simulink library "carnot"  (R2018b)
settings: Solver=VariableStepAuto  StartTime=0.0  StopTime=10.0  RelTol=1e-3
undefined symbols (not defined in the file or in its folder): A, A_earth, acol, Acol, ActPower1, ActPower2, ActPower3, Ad, Ad0, Ar, Au, Au0, Azimuth_Angle, B, Bd, Bd0, Br, Bu, Bu0, C, c1, c2, c3, c33, c4, c5, c6, CarnotCallbacks_Density, CarnotCallbacks_Enthalpy, CarnotCallbacks_Enthalpy2Temperature, CarnotCallbacks_Entropy, CarnotCallbacks_Evaporation_Enthalpy, CarnotCallbacks_GlobalMessageLevel, CarnotCallbacks_Grashof, CarnotCallbacks_Heat_Capacity, CarnotCallbacks_Kinematic_Viscosity, CarnotCallbacks_PMV_PPD, CarnotCallbacks_Prandtl, CarnotCallbacks_Saturation_Property, CarnotCallbacks_Saturation_Temperature, CarnotCallbacks_Saturation_Value_Water, CarnotCallbacks_Specific_Volume, CarnotCallbacks_Thermal_Conductivity, CarnotCallbacks_Vapour_Content, CarnotCallbacks_Vapour_Pressure, Cd, Cdl, Cr, Cu, Davies, Dd, DE_TRY2010_04_averageYear, delta_grd, density, DiameterLastPiece, dl, DPConstant, DPLinear, DPQuadratic, Dr ... (+59)
libraries: $bdroot x429, simulink x36, simulink_extras x12
(part 13 of 22)

== system carnot/Basic/Hydraulics/Grashof ==
  Twall : Inport
  Tinf : Inport  Port=2
  p : Inport  Port=3
  Fluid_Type : Inport  Port=4
  Fluid_Mix : Inport  Port=5
  dimension : Inport  Port=6
  SFunction : S-Function  FunctionName=grashofn  Parameters=DEBUGLEVEL,MAXTOTALMESSAGES,MAXCONSECUTIVEMESSAGES,WRITETOFILE,FILENAME  SFunctionDeploymentMode=off  EnableBusSupport=off
  Gr : Outport
  wires:
  SFunction/1 -> Gr/1
  Fluid_Type/1 -> SFunction/1
  Fluid_Mix/1 -> SFunction/2
  Twall/1 -> SFunction/3
  Tinf/1 -> SFunction/4
  p/1 -> SFunction/5
  dimension/1 -> SFunction/6

== system carnot/Basic/Hydraulics/Mix_T_Mdot ==
  THB1 : Inport
  THB2 : Inport  Port=2
  Add : Sum
  Bus Selector2 : BusSelector  OutputSignals=MassFlow
  Bus Selector3 : BusSelector  OutputSignals=MassFlow
  S-Function : S-Function  FunctionName=mix_temperature  Parameters=mixcalc  SFunctionDeploymentMode=off  EnableBusSupport=off
  select1 : Subsystem
  select2 : Subsystem
  T : Outport
  mdot : Outport  Port=2
  mix : Outport  Port=3
  wires:
  select2/1(Out1) -> S-Function/2
  select1/1(Out1) -> S-Function/1
  S-Function/1 -> T/1  "T"
  THB2/1 -> select2/1(In1), Bus Selector3/1
  S-Function/2 -> mix/1  "mix"
  THB1/1 -> select1/1(In1), Bus Selector2/1
  Bus Selector3/1 -> Add/2  "<MassFlow>"
  Bus Selector2/1 -> Add/1  "<MassFlow>"
  Add/1 -> mdot/1

== system carnot/Basic/Hydraulics/Prandtl ==
  T : Inport
  p : Inport  Port=2
  Fluid_Type : Inport  Port=3
  Fluid_Mix : Inport  Port=4
  SFunction : S-Function  FunctionName=prandtln  Parameters=DEBUGLEVEL,MAXTOTALMESSAGES,MAXCONSECUTIVEMESSAGES,WRITETOFILE,FILENAME  SFunctionDeploymentMode=off  EnableBusSupport=off
  Pr : Outport
  wires:
  SFunction/1 -> Pr/1
  T/1 -> SFunction/3
  p/1 -> SFunction/4
  Fluid_Type/1 -> SFunction/1
  Fluid_Mix/1 -> SFunction/2

== system carnot/Basic/Hydraulics/Reynolds ==
  T : Inport
  v : Inport  Port=2
  p : Inport  Port=3
  "fluid, mix" : Inport  Port=4
  dimension : Inport  Port=5
  Demux1 : Demux  Outputs=2
  Kinematic_Viscosity : $bdroot/Basic/Material_Properties/Kinematic_Viscosity  VariantControl=CarlibClassic  INPUTARGUMENTS=state variables (classic)  DEBUGLEVEL=WARNINGLEVEL  MAXTOTALMESSAGES=inf  MAXCONSECUTIVEMESSAGES=inf  WRITETOFILE=0  FILENAME='errors.txt'
  Product : Product  Inputs=/**  SaturateOnIntegerOverflow=on  InputSameDT=on  OutDataTypeStr=Inherit: Same as first input
  Re : Outport
  wires:
  Product/1 -> Re/1
  v/1 -> Product/2
  dimension/1 -> Product/3
  p/1 -> Kinematic_Viscosity/2
  T/1 -> Kinematic_Viscosity/1
  Demux1/1 -> Kinematic_Viscosity/3
  "fluid, mix"/1 -> Demux1/1
  Kinematic_Viscosity/1 -> Product/1
  Demux1/2 -> Kinematic_Viscosity/4

== system carnot/Basic/Hydraulics/ReynoldsTHB ==
  THB : Inport
  Diameter : Inport  Port=2
  Bus Selector : BusSelector  OutputSignals=Temperature,MassFlow,Pressure
  Bus Selector1 : BusSelector  OutputSignals=FluidType,FluidMix  OutputAsBus=on
  Bus Selector2 : BusSelector  OutputSignals=Temperature,Pressure
  Bus Selector3 : BusSelector  OutputSignals=FluidType,FluidMix  OutputAsBus=on
  Reynolds1 : $bdroot/Basic/Hydraulics/Reynolds
  Terminator : Terminator
  Velocity1 : $bdroot/Basic/Hydraulics/Velocity
  Re : Outport
  wires:
  Velocity1/1 -> Reynolds1/2
  Bus Selector/2 -> Velocity1/2  "<MassFlow>"
  Bus Selector/1 -> Velocity1/1  "<Temperature>"
  Bus Selector/3 -> Velocity1/3  "<Pressure>"
  Bus Selector1/1 -> Velocity1/4
  Bus Selector2/1 -> Reynolds1/1  "<Temperature>"
  Bus Selector3/1 -> Reynolds1/4
  Bus Selector2/2 -> Reynolds1/3  "<Pressure>"
  Velocity1/2 -> Terminator/1
  THB/1 -> Bus Selector/1, Bus Selector1/1, Bus Selector2/1, Bus Selector3/1
  Reynolds1/1 -> Re/1
  Diameter/1 -> Velocity1/5, Reynolds1/5

== system carnot/Basic/Hydraulics/THBCreator ==
  ID : Inport
  Temperature : Inport  Port=2
  MassFlow : Inport  Port=3
  Pressure : Inport  Port=4
  FluidType : Inport  Port=5
  FluidMix : Inport  Port=6
  FluidMix2 : Inport  Port=7
  FluidMix3 : Inport  Port=8
  DiameterLastPiece : Inport  Port=9
  DPConstant : Inport  Port=10
  DPLinear : Inport  Port=11
  DPQuadratic : Inport  Port=12
  HydraulicInductance : Inport  Port=13
  GeodeticHeight : Inport  Port=14
  BusCreator : BusCreator  Inputs=14  OutDataTypeStr=Bus: THB
  THB : Outport  OutDataTypeStr=Bus: THB
  wires:
  BusCreator/1 -> THB/1
  ID/1 -> BusCreator/1  "ID"
  Temperature/1 -> BusCreator/2  "Temperature"
  MassFlow/1 -> BusCreator/3  "MassFlow"
  Pressure/1 -> BusCreator/4  "Pressure"
  FluidType/1 -> BusCreator/5  "FluidType"
  FluidMix/1 -> BusCreator/6  "FluidMix"
  FluidMix2/1 -> BusCreator/7  "FluidMix2"
  FluidMix3/1 -> BusCreator/8  "FluidMix3"
  DiameterLastPiece/1 -> BusCreator/9  "DiameterLastPiece"
  DPConstant/1 -> BusCreator/10  "DPConstant"
  DPLinear/1 -> BusCreator/11  "DPLinear"
  DPQuadratic/1 -> BusCreator/12  "DPQuadratic"
  HydraulicInductance/1 -> BusCreator/13  "HydraulicInductance"
  GeodeticHeight/1 -> BusCreator/14  "GeodeticHeight"

== system carnot/Basic/Hydraulics/Velocity ==
  T : Inport
  mdot : Inport  Port=2
  p : Inport  Port=3
  "fluid, mix" : Inport  Port=4
  d : Inport  Port=5
  Demux1 : Demux  Outputs=2
  Density : $bdroot/Basic/Material_Properties/Density  VariantControl=CarlibClassic  INPUTARGUMENTS=state variables (classic)  DEBUGLEVEL=DEBUGLEVEL  MAXTOTALWARNINGS=inf  MAXCONSECUTIVEWARNINGS=inf  WRITETOFILE=0  FILENAME='errors.txt'
  Math Function : Math  Operator=square  SaturateOnIntegerOverflow=on
  Product : Product  Inputs=*//  SaturateOnIntegerOverflow=on  InputSameDT=on  OutDataTypeStr=Inherit: Same as first input
  quadratic : Gain  Gain=pi/4  SaturateOnIntegerOverflow=on  OutDataTypeStr=Inherit: Same as input  ParamDataTypeStr=Inherit: Same as input
  v : Outport
  density : Outport  Port=2
  wires:
  p/1 -> Density/2
  "fluid, mix"/1 -> Demux1/1
  Demux1/1 -> Density/3
  mdot/1 -> Product/1
  Demux1/2 -> Density/4
  T/1 -> Density/1
  Product/1 -> v/1
  d/1 -> Math Function/1
  Math Function/1 -> quadratic/1
  quadratic/1 -> Product/2
  Density/1 -> Product/3, density/1

== system carnot/Basic/Hydraulics/basic_THB ==
  Bus Creator : BusCreator  InitFcn=load THB.mat  Inputs=14  OutDataTypeStr=Bus: THB
  const1 : Constant  Value=hgt
  const2 : Constant  Value=mix2
  const21 : Constant  Value=ID  mask{mID=Pressure Drop from Massflow}
      mask prompts: mID "ID for pressure drop calculation"
      mask init:
      | ID = (mID-1)*10000+1;
      mask TypeOptions mID: No Pressure Drop | Pressure Drop from Massflow | Full Pressure Drop with Static Height
  const{22..23,30..31} (4 alike) : Constant  Value=0
  const24 : Constant  Value=t
  const25 : Constant  Value=mdot
  const26 : Constant  Value=p
  const27 : Constant  Value=fluid  mask{fluid=Water}
      mask TypeOptions fluid: Water | Air | Cotton Oil | Silicone Oil | Water-Glycol Mix | Tyfocor LS | Water (Constant 20°C) | Air (dry+ constant 20°C)
  const28 : Constant  Value=mix
  const29 : Constant  Value=dia
  const3 : Constant  Value=mix3
  THB : Outport
  wires:
  const28/1 -> Bus Creator/6  "FluidMix"
  const27/1 -> Bus Creator/5  "FluidType"
  const26/1 -> Bus Creator/4  "Pressure"
  const25/1 -> Bus Creator/3  "MassFlow"
  const24/1 -> Bus Creator/2  "Temperature"
  const21/1 -> Bus Creator/1  "ID"
  Bus Creator/1 -> THB/1
  const30/1 -> Bus Creator/10  "DPConstant"
  const29/1 -> Bus Creator/9  "DiameterLastPiece"
  const22/1 -> Bus Creator/11  "DPLinear"
  const23/1 -> Bus Creator/12  "DPQuadratic"
  const31/1 -> Bus Creator/13  "HydraulicInductance"
  const1/1 -> Bus Creator/14  "GeodeticHeight"
  const2/1 -> Bus Creator/7  "FluidMix2"
  const3/1 -> Bus Creator/8  "FluidMix3"

== system carnot/Basic/Hydraulics/basic_create_THB ==
  mdot : Inport
  T : Inport  Port=2
  THB_set_T : $bdroot/Source/Simple/THB_set_T
  THB_set_mdot : $bdroot/Source/Simple/THB_set_mdot
  basic_THB : $bdroot/Basic/Hydraulics/basic_THB  t=10  mdot=0  p=p  ID=No Pressure Drop  fluid=Water  mix=mix  mix2=mix2  mix3=mix3  dia=dia  hgt=hgt
  THB : Outport
  wires:
  T/1 -> THB_set_T/2
  THB_set_T/1 -> THB/1
  THB_set_mdot/1 -> THB_set_T/1
  mdot/1 -> THB_set_mdot/2
  basic_THB/1 -> THB_set_mdot/1

== system carnot/Basic/Material_Properties/AIV_WetBulbTemperature ==
  AIV : Inport
  AIV_selector : $bdroot/Outputs/AIV_selector  e1=off  e2=on  e3=off  e4=off  e5=off  e6=off  e7=off  e8=off  e9=off
  AIV_selector1 : $bdroot/Outputs/AIV_selector  e1=off  e2=off  e3=off  e4=off  e5=off  e6=off  e7=off  e8=on  e9=off
  AIV_selector2 : $bdroot/Outputs/AIV_selector  e1=off  e2=off  e3=off  e4=on  e5=off  e6=off  e7=off  e8=off  e9=off
  Bus Assignment : BusAssignment  AssignedSignals=Temperature,Pressure,FluidMix
  Constant_THB : $bdroot/Source/Simple/Constant_THB  t=20  mdot=0  p=1e5  mID=No Pressure Drop  fluid=Air  mix=0  mix2=0  mix3=0  dia=0.02  hgt=0
  THB_WetBulbTemperature : $bdroot/Basic/Material_Properties/THB_WetBulbTemperature
  WBT : Outport
  rel_hum : Outport  Port=2
  wires:
  THB_WetBulbTemperature/2 -> rel_hum/1
  Bus Assignment/1 -> THB_WetBulbTemperature/1
  Constant_THB/1 -> Bus Assignment/1
  AIV_selector1/1 -> Bus Assignment/3  "p"
  AIV_selector2/1 -> Bus Assignment/4  "mix"
  AIV_selector/1 -> Bus Assignment/2  "T"
  AIV/1 -> AIV_selector/1, AIV_selector2/1, AIV_selector1/1
  THB_WetBulbTemperature/1 -> WBT/1

== system carnot/Basic/Material_Properties/Density ==
  T : Inport
  p : Inport  Port=2
  Fluid_Type : Inport  Port=3
  Fluid_Mix : Inport  Port=4
  SFunction : S-Function  FunctionName=rhofluid  Parameters=DEBUGLEVEL-1,MAXTOTALWARNINGS,MAXCONSECUTIVEWARNINGS,WRITETOFILE,FILENAME  SFunctionDeploymentMode=off  EnableBusSupport=off
  density : Outport
  wires:
  SFunction/1 -> density/1
  T/1 -> SFunction/3
  p/1 -> SFunction/4
  Fluid_Type/1 -> SFunction/1
  Fluid_Mix/1 -> SFunction/2

== system carnot/Basic/Material_Properties/Enthalpy ==
  T : Inport
  p : Inport  Port=2
  Fluid_Type : Inport  Port=3
  Fluid_Mix : Inport  Port=4
  SFunction : S-Function  FunctionName=enthaflu  Parameters=DEBUGLEVEL,MAXTOTALMESSAGES,MAXCONSECUTIVEMESSAGES,WRITETOFILE,FILENAME  SFunctionDeploymentMode=off  EnableBusSupport=off
  enthalpy : Outport
  wires:
  SFunction/1 -> enthalpy/1
  T/1 -> SFunction/3
  p/1 -> SFunction/4
  Fluid_Type/1 -> SFunction/1
  Fluid_Mix/1 -> SFunction/2

== system carnot/Basic/Material_Properties/Enthalpy2Temperature ==
  enthalpy : Inport
  p : Inport  Port=2
  Fluid_Type : Inport  Port=3
  Fluid_Mix : Inport  Port=4
  SFunction : S-Function  FunctionName=enth2temp  Parameters=DEBUGLEVEL,MAXTOTALMESSAGES,MAXCONSECUTIVEMESSAGES,WRITETOFILE,FILENAME  SFunctionDeploymentMode=off  EnableBusSupport=off
  T : Outport
  wires:
  SFunction/1 -> T/1
  Fluid_Type/1 -> SFunction/1
  Fluid_Mix/1 -> SFunction/2
  enthalpy/1 -> SFunction/3
  p/1 -> SFunction/4

== system carnot/Basic/Material_Properties/Entropy ==
  T : Inport
  p : Inport  Port=2
  Fluid_Type : Inport  Port=3
  Fluid_Mix : Inport  Port=4
  SFunction : S-Function  FunctionName=entroflu  Parameters=DEBUGLEVEL,MAXTOTALMESSAGES,MAXCONSECUTIVEMESSAGES,WRITETOFILE,FILENAME  SFunctionDeploymentMode=off  EnableBusSupport=off
  entropy : Outport
  wires:
  SFunction/1 -> entropy/1
  T/1 -> SFunction/3
  p/1 -> SFunction/4
  Fluid_Type/1 -> SFunction/1
  Fluid_Mix/1 -> SFunction/2

== system carnot/Basic/Material_Properties/Evaporation_Enthalpy ==
  T : Inport
  p : Inport  Port=2
  Fluid_Type : Inport  Port=3
  Fluid_Mix : Inport  Port=4
  SFunction : S-Function  FunctionName=evapoent  Parameters=DEBUGLEVEL,MAXTOTALMESSAGES,MAXCONSECUTIVEMESSAGES,WRITETOFILE,FILENAME  SFunctionDeploymentMode=off  EnableBusSupport=off
  evap_enthalpy : Outport
  wires:
  SFunction/1 -> evap_enthalpy/1
  T/1 -> SFunction/3
  p/1 -> SFunction/4
  Fluid_Type/1 -> SFunction/1
  Fluid_Mix/1 -> SFunction/2

== system carnot/Basic/Material_Properties/Heat_Capacity ==
  T : Inport
  p : Inport  Port=2
  Fluid_Type : Inport  Port=3
  Fluid_Mix : Inport  Port=4
  SFunction : S-Function  FunctionName=capfluid  Parameters=DEBUGLEVEL-1,MAXTOTALWARNINGS,MAXCONSECUTIVEWARNINGS,WRITETOFILE,FILENAME  SFunctionDeploymentMode=off  EnableBusSupport=off
  cp : Outport
  wires:
  SFunction/1 -> cp/1
  T/1 -> SFunction/3
  p/1 -> SFunction/4
  Fluid_Type/1 -> SFunction/1
  Fluid_Mix/1 -> SFunction/2

== system carnot/Basic/Material_Properties/Input_Air ==
  Fluid_mix : Constant  Value=x
  Fluid_type : Constant  Value=2
  Temp : Constant  Value=T
  pres : Constant  Value=p
  Temperature : Outport
  Pressure : Outport  Port=2
  Fluid_type: air : Outport  Port=3
  absolute_humidity : Outport  Port=4
  wires:
  Fluid_mix/1 -> absolute_humidity/1
  Fluid_type/1 -> Fluid_type: air/1
  Temp/1 -> Temperature/1
  pres/1 -> Pressure/1

== system carnot/Basic/Material_Properties/Input_Cotton_Oil ==
  Fluid_mix : Constant  Value=0
  Fluid_type : Constant  Value=3
  Temp : Constant  Value=T
  pres : Constant  Value=p
  Temperature : Outport
  Pressure : Outport  Port=2
  Fluid_cotton_oil : Outport  Port=3
  mix : Outport  Port=4
  wires:
  pres/1 -> Pressure/1
  Temp/1 -> Temperature/1
  Fluid_type/1 -> Fluid_cotton_oil/1
  Fluid_mix/1 -> mix/1

== system carnot/Basic/Material_Properties/Input_Fluid ==
  Fluid_mix_ : Constant  Value=x
  Fluid_type_ : Constant  Value=fluid
  Temp : Constant  Value=T
  pres : Constant  Value=p
  Temperature : Outport
  Pressure : Outport  Port=2
  Fluid_type : Outport  Port=3
  Fluid_mix : Outport  Port=4
  wires:
  pres/1 -> Pressure/1
  Temp/1 -> Temperature/1
  Fluid_type_/1 -> Fluid_type/1
  Fluid_mix_/1 -> Fluid_mix/1

== system carnot/Basic/Material_Properties/Input_Silicon_Oil ==
  Fluid_mix : Constant  Value=0
  Fluid_type : Constant  Value=4
  Temp : Constant  Value=T
  pres : Constant  Value=p
  Temperature : Outport
  Pressure : Outport  Port=2
  Fluid_silicon_oil : Outport  Port=3
  mix : Outport  Port=4
  wires:
  Fluid_mix/1 -> mix/1
  Fluid_type/1 -> Fluid_silicon_oil/1
  Temp/1 -> Temperature/1
  pres/1 -> Pressure/1

== system carnot/Basic/Material_Properties/Input_Tyfocor_LS ==
  Fluid_mix : Constant  Value=0
  Fluid_type : Constant  Value=6
  Temp : Constant  Value=T
  pres : Constant  Value=p
  Temperature : Outport
  Pressure : Outport  Port=2
  Fluid_TyfocorLS : Outport  Port=3
  mix : Outport  Port=4
  wires:
  pres/1 -> Pressure/1
  Temp/1 -> Temperature/1
  Fluid_type/1 -> Fluid_TyfocorLS/1
  Fluid_mix/1 -> mix/1

== system carnot/Basic/Material_Properties/Input_Water ==
  Fluid_mix : Constant  Value=xd
  Fluid_type : Constant
  Temp : Constant  Value=T
  pres : Constant  Value=p
  Temperature : Outport
  Pressure : Outport  Port=2
  Fluid_type: water : Outport  Port=3
  vapour_content : Outport  Port=4
  wires:
  pres/1 -> Pressure/1
  Temp/1 -> Temperature/1
  Fluid_type/1 -> Fluid_type: water/1
  Fluid_mix/1 -> vapour_content/1

== system carnot/Basic/Material_Properties/Input_Water_Glycol ==
  Fluid_mix : Constant  Value=g
  Fluid_type : Constant  Value=5
  Temp : Constant  Value=T
  pres : Constant  Value=p
  Temperature : Outport
  Pressure : Outport  Port=2
  Fluid_type: water/glycol : Outport  Port=3
  "volume content of glycol " : Outport  Port=4
  wires:
  pres/1 -> Pressure/1
  Temp/1 -> Temperature/1
  Fluid_type/1 -> Fluid_type: water/glycol/1
  Fluid_mix/1 -> "volume content of glycol "/1

== system carnot/Basic/Material_Properties/Kinematic_Viscosity ==
  T : Inport
  p : Inport  Port=2
  Fluid_Type : Inport  Port=3
  Fluid_Mix : Inport  Port=4
  SFunction : S-Function  FunctionName=viscous  Parameters=DEBUGLEVEL,MAXTOTALMESSAGES,MAXCONSECUTIVEMESSAGES,WRITETOFILE,FILENAME  SFunctionDeploymentMode=off  EnableBusSupport=off
  visc : Outport
  wires:
  SFunction/1 -> visc/1
  T/1 -> SFunction/3
  p/1 -> SFunction/4
  Fluid_Type/1 -> SFunction/1
  Fluid_Mix/1 -> SFunction/2

== system carnot/Basic/Material_Properties/PhaseCheck ==
  THBin : Inport
  S-Function : S-Function  FunctionName=phasechk  SFunctionDeploymentMode=off  EnableBusSupport=off
  Selector : Selector  InputPortWidth=20  IndexOptions=Index vector (dialog)  Indices=[2:6]  OutputSizes=1
  THB2THV : $bdroot/Toolbox/THB2THV
  wires:
  Selector/1 -> S-Function/1
  THBin/1 -> THB2THV/1
  THB2THV/1 -> Selector/1

== system carnot/Basic/Material_Properties/RelHum2x ==
  note: RG      f · ps
      |  x  = ----  --------------
      |         RD     p - f · ps
      |
      | RG = 287.1 Nm/kgK (Gas Constant Air)
      | RD = 461.5 Nm/kgK (Gas Constant Water Vapour)
      | x absolute Humudity
      | f relative Humidity
      | pD partial pressure of water vapour
  T : Inport
  p : Inport  Port=2
  rel_hum : Inport  Port=3
  Product : Product  Inputs=*/  SaturateOnIntegerOverflow=on  InputSameDT=on  OutDataTypeStr=Inherit: Same as first input
  Product1 : Product  Inputs=*/  SaturateOnIntegerOverflow=on  InputSameDT=on  OutDataTypeStr=Inherit: Same as first input
  Saturation : Saturate  UpperLimit=inf  LowerLimit=0
  Sum : Sum  Inputs=-+  SaturateOnIntegerOverflow=on  InputSameDT=on  OutDataTypeStr=Inherit: Same as first input
  Vapour_Pressure : $bdroot/Basic/Material_Properties/Vapour_Pressure  VariantControl=CarlibClassic  INPUTARGUMENTS=state variables (classic)  DEBUGLEVEL=WARNINGLEVEL  MAXTOTALMESSAGES=inf  MAXCONSECUTIVEMESSAGES=inf  WRITETOFILE=0  FILENAME='errors.txt'
  mix : Constant  Value=0
  molar mass fraction : Gain  Gain=287.1/461.5  SaturateOnIntegerOverflow=on  OutDataTypeStr=Inherit: Same as input  ParamDataTypeStr=Inherit: Same as input
  p12 : Constant
  percent2absolute : Gain  Gain=0.01  SaturateOnIntegerOverflow=on  OutDataTypeStr=Inherit: Same as input  ParamDataTypeStr=Inherit: Same as input
  water : Constant
  x : Outport
  wires:
  p/1 -> Product/1
  Product/1 -> Sum/2
  Sum/1 -> Product1/2
  Product1/1 -> molar mass fraction/1
  T/1 -> Vapour_Pressure/1
  water/1 -> Vapour_Pressure/3
  p12/1 -> Vapour_Pressure/2
  mix/1 -> Vapour_Pressure/4
  Vapour_Pressure/1 -> Sum/1, Product1/1
  rel_hum/1 -> percent2absolute/1
  percent2absolute/1 -> Product/2
  molar mass fraction/1 -> Saturation/1
  Saturation/1 -> x/1

== system carnot/Basic/Material_Properties/Saturation_Property ==
  T : Inport
  p : Inport  Port=2
  Fluid_Type : Inport  Port=3
  Fluid_Mix : Inport  Port=4
  SFunction : S-Function  FunctionName=satprop  Parameters=PROPERTY, FLUIDPHASE, DEBUGLEVEL, MAXTOTALMESSAGES, MAXCONSECUTIVEMESSAGES, WRITETOFILE, FILENAME  SFunctionDeploymentMode=off  EnableBusSupport=off
  satprop : Outport
  wires:
  SFunction/1 -> satprop/1
  T/1 -> SFunction/3
  p/1 -> SFunction/4
  Fluid_Type/1 -> SFunction/1
  Fluid_Mix/1 -> SFunction/2

== system carnot/Basic/Material_Properties/Saturation_Temperature ==
  T : Inport
  p : Inport  Port=2
  Fluid_Type : Inport  Port=3
  Fluid_Mix : Inport  Port=4
  SFunction : S-Function  FunctionName=satutemp  Parameters=DEBUGLEVEL,MAXTOTALMESSAGES,MAXCONSECUTIVEMESSAGES,WRITETOFILE,FILENAME  SFunctionDeploymentMode=off  EnableBusSupport=off
  Tsat : Outport
  wires:
  SFunction/1 -> Tsat/1
  T/1 -> SFunction/3
  p/1 -> SFunction/4
  Fluid_Type/1 -> SFunction/1
  Fluid_Mix/1 -> SFunction/2

== system carnot/Basic/Material_Properties/Saturation_Value_Water ==
  T : Inport
  p : Inport  Port=2
  Fluid_Type : Inport  Port=3
  Fluid_Mix : Inport  Port=4
  property_id : Inport  Port=5
  SFunction : S-Function  FunctionName=satprop_vec  Parameters=DEBUGLEVEL,MAXTOTALMESSAGES,MAXCONSECUTIVEMESSAGES,WRITETOFILE,FILENAME  SFunctionDeploymentMode=off  EnableBusSupport=off
  saturation_vapour : Outport
  saturation_liquid : Outport  Port=2
  wires:
  SFunction/1 -> saturation_vapour/1
  SFunction/2 -> saturation_liquid/1
  T/1 -> SFunction/3
  p/1 -> SFunction/4
  Fluid_Type/1 -> SFunction/1
  Fluid_Mix/1 -> SFunction/2
  property_id/1 -> SFunction/5

== system carnot/Basic/Material_Properties/Specific_Volume ==
  T : Inport
  p : Inport  Port=2
  Fluid_Type : Inport  Port=3
  Fluid_Mix : Inport  Port=4
  SFunction : S-Function  FunctionName=specivol  Parameters=DEBUGLEVEL-1,MAXTOTALWARNINGS,MAXCONSECUTIVEWARNINGS,WRITETOFILE,FILENAME  SFunctionDeploymentMode=off  EnableBusSupport=off
  spec_vol : Outport
  wires:
  SFunction/1 -> spec_vol/1
  T/1 -> SFunction/3
  p/1 -> SFunction/4
  Fluid_Type/1 -> SFunction/1
  Fluid_Mix/1 -> SFunction/2

== system carnot/Basic/Material_Properties/THB_WetBulbTemperature ==
  THB_air : Inport
  Bus Selector : BusSelector  OutputSignals=Temperature,Pressure,FluidType,FluidMix
  Compare To Constant : simulink/Logic and Bit Operations/Compare To Constant  relop===  const=2  OutDataTypeStr=uint8  ZeroCross=off
  Constant : Constant
  Gain : Gain  Gain=100
  MinMax : MinMax  Inputs=2
  Product : Product  Inputs=*/  RndMeth=Zero
  Product1 : Product  RndMeth=Zero
  Product2 : Product  RndMeth=Zero
  Saturation : Saturate  UpperLimit=100  LowerLimit=0
  Vapour_Pressure1 : $bdroot/Basic/Material_Properties/Vapour_Pressure  VariantControl=CarlibClassic  INPUTARGUMENTS=state variables (classic)  DEBUGLEVEL=WARNINGLEVEL  MAXTOTALMESSAGES=inf  MAXCONSECUTIVEMESSAGES=inf  WRITETOFILE=0  FILENAME='errors.txt'
  Vapour_Pressure2 : $bdroot/Basic/Material_Properties/Vapour_Pressure  VariantControl=CarlibClassic  INPUTARGUMENTS=state variables (classic)  DEBUGLEVEL=WARNINGLEVEL  MAXTOTALMESSAGES=inf  MAXCONSECUTIVEMESSAGES=inf  WRITETOFILE=0  FILENAME='errors.txt'
  WBT Fcn of relHum+DBT : Lookup2D  RowIndex=[0,5,10,15,20,25,30,35,40,45,50,55,60,65,70,75,80,85,90,95,100]  ColumnIndex=[-6,-4,-2,0,2,4,6,8,10,12,14,16,18,20,22,24,26,28,30,32,34,36,38,40]  Table=reshape([-10.3,-10.1,-9.9,-9.3,-9.3,-8.9,-8.8,-8.8,-8.3,-8.2,-8.2,-7.7,-7.7,-7.7,-7.1,-7.1,-7.1,-6.6,-6.6,-6.0,-6,-8.3,-8.1,-7.9,-7.9,-7.8,-7.3,-7.3,-6.8,-6.8,-6.7,-6.2,-6.2,-5.7,-5.7,-5.6,-5.1,-5.1,-4.6,-4.6,-4.6,-4,-7.2,-6.9,-6.7,-6.4,-6.1,-5.9,-5.6,-5.3,-5.0,-4.8,-4.8,-4.2,-4.2,-3.7,-3.7,-3.1,-3.1,-2.6,-2.6,-2.6,-2,-5.6,-5.3,-5.0,-5.0,-4.4,-4.4,-3.9,-3.9,-3.3,-3.3,-2.8,-2.8,-2.2,-2.2,-1.7,-1.7,-1.1,-1.1,-0.6,-0.6,0,-4.5,-4.2,-3.9,-3.6,-3.0,-2.8,-2.4,-1.9,-1.9,-1.3,-1.3,-0.8,-0.6,-0.2,0.1,0.4,0.7,1.1,1.4,1.7,2,-3.4,-3.0,-2.7,-2.1,-1.6,-1.1,-1.0,-0.4,0.0,0.1,0.5,0.8,1.2,1.6,1.9,2.3,2.6,3.0,3.3,3.7,4,-1.9,-1.5,-1.1,-0.7,-0.3,0.1,0.5,0.9,1.3,1.8,2.2,2.6,3.0,3.4,3.8,4.1,4.5,4.9,5.3,5.6,6,-0.8,-0.4,0.1,0.6,1.1,1.5,2.0,2.5,2.9,3.4,3.8,4.3,4.7,5.1,5.6,6.0,6.4,6.8,7.2,7.6,8,0.3,0.8,1.4,1.9,2.5,3.0,3.5,4.0,4.5,5.0,5.5,6.0,6.5,6.9,7.4,7.8,8.3,8.7,9.2,9.6,10,1.4,2.1,2.7,3.3,3.9,4.4,5.0,5.6,6.1,6.6,7.2,7.7,8.2,8.7,9.2,9.7,10.2,10.6,11.1,11.6,12,2.6,3.2,3.9,4.6,5.2,5.8,6.5,7.1,7.7,8.2,8.8,9.4,9.9,10.5,11.0,11.5,12.0,12.5,13.0,13.5,14,3.7,4.4,5.1,5.9,6.6,7.3,7.9,8.6,9.2,9.9,10.5,11.1,11.7,12.2,12.8,13.4,13.9,14.5,15.0,15.5,16,4.7,5.5,6.3,7.1,7.9,8.6,9.4,10.1,10.8,11.5,12.1,12.8,13.4,14.0,14.6,15.2,15.8,16.4,16.9,17.5,18,5.7,6.6,7.5,8.4,9.2,10.0,10.8,11.6,12.3,13.1,13.8,14.5,15.1,15.8,16.4,17.1,17.7,18.3,18.9,19.4,20,6.7,7.7,8.7,9.6,10.5,11.4,12.2,13.1,13.9,14.6,15.4,16.1,16.9,17.6,18.2,18.9,19.6,20.2,20.8,21.4,22,7.7,8.8,9.8,10.8,11.8,12.8,13.7,14.6,15.4,16.2,17.0,17.8,18.6,19.3,20.1,20.8,21.4,22.1,22.7,23.4,24,8.6,9.8,11.0,12.1,13.1,14.1,15.1,16.0,17.0,17.8,18.7,19.5,20.3,21.1,21.9,22.6,23.3,24.0,24.7,25.4,26,9.6,10.8,12.1,13.3,14.4,15.5,16.5,17.5,18.5,19.4,20.3,21.2,22.1,22.9,23.7,24.5,25.2,25.9,26.6,27.3,28,10.4,11.8,13.2,14.4,15.7,16.8,17.9,19.0,20.0,21.0,22.0,22.9,23.8,24.7,25.5,26.3,27.1,27.8,28.6,29.3,30,11.3,12.8,14.3,15.6,16.9,18.2,19.4,20.5,21.6,22.6,23.6,24.6,25.5,26.4,27.3,28.2,29.0,29.8,30.5,31.3,32,12.1,13.8,15.3,16.8,18.2,19.5,20.8,22.0,23.1,24.2,25.3,26.3,27.3,28.2,29.1,30.0,30.9,31.7,32.5,33.3,34,12.9,14.7,16.4,18.0,19.5,20.9,22.2,23.5,24.7,25.9,27.0,28.0,29.0,30.0,31.0,31.9,32.8,33.6,34.4,35.2,36,13.7,15.7,17.5,19.1,20.7,22.2,23.6,25.0,26.3,27.5,28.6,29.7,30.8,31.8,32.8,33.7,34.7,35.5,36.4,37.2,38,14.5,16.6,18.5,20.3,22.0,23.6,25.1,26.5,27.8,29.1,30.3,31.5,32.6,33.6,34.6,35.6,36.6,37.5,38.3,39.2,40],21,24)  RndMeth=Nearest  LUTDesignDataSource=Matlab Workspace  LUTDesignUseExistingBP=off  LUTDesignAbsError=NaN
  WBT : Outport
  rel_hum : Outport  Port=2
  wires:
  Compare To Constant/1 -> Product1/2, Product2/2
  Product2/1 -> WBT/1
  Product1/1 -> rel_hum/1
  Saturation/1 -> Product1/1, WBT Fcn of relHum+DBT/1
  Gain/1 -> Saturation/1
  WBT Fcn of relHum+DBT/1 -> Product2/1
  Product/1 -> Gain/1
  MinMax/1 -> Product/1
  Vapour_Pressure2/1 -> Product/2, MinMax/2
  Vapour_Pressure1/1 -> MinMax/1
  Constant/1 -> Vapour_Pressure2/3, Vapour_Pressure2/4
  Bus Selector/1 -> Vapour_Pressure1/1, Vapour_Pressure2/1, WBT Fcn of relHum+DBT/2  "<Temperature>"
  Bus Selector/4 -> Vapour_Pressure1/4  "<FluidMix>"
  Bus Selector/3 -> Compare To Constant/1, Vapour_Pressure1/3  "<FluidType>"
  Bus Selector/2 -> Vapour_Pressure1/2, Vapour_Pressure2/2  "<Pressure>"
  THB_air/1 -> Bus Selector/1

== system carnot/Basic/Material_Properties/Temperature_Conductivity ==
  T : Inport
  p : Inport  Port=2
  Fluid_Type : Inport  Port=3
  Fluid_Mix : Inport  Port=4
  SFunction : S-Function  FunctionName=tempconduct  Parameters=DEBUGLEVEL,MAXTOTALMESSAGES,MAXCONSECUTIVEMESSAGES,WRITETOFILE,FILENAME  SFunctionDeploymentMode=off  EnableBusSupport=off
  Tcond : Outport
  wires:
  SFunction/1 -> Tcond/1
  T/1 -> SFunction/3
  p/1 -> SFunction/4
  Fluid_Type/1 -> SFunction/1
  Fluid_Mix/1 -> SFunction/2

== system carnot/Basic/Material_Properties/Thermal_Conductivity ==
  T : Inport
  p : Inport  Port=2
  Fluid_Type : Inport  Port=3
  Fluid_Mix : Inport  Port=4
  SFunction : S-Function  FunctionName=conduct  Parameters=DEBUGLEVEL,MAXTOTALMESSAGES,MAXCONSECUTIVEMESSAGES,WRITETOFILE,FILENAME  SFunctionDeploymentMode=off  EnableBusSupport=off
  cond : Outport
  wires:
  SFunction/1 -> cond/1
  T/1 -> SFunction/3
  p/1 -> SFunction/4
  Fluid_Type/1 -> SFunction/1
  Fluid_Mix/1 -> SFunction/2

== system carnot/Basic/Material_Properties/Vapour_Content ==
  T : Inport
  p : Inport  Port=2
  Fluid_Type : Inport  Port=3
  Fluid_Mix : Inport  Port=4
  value : Inport  Port=5
  SFunction : S-Function  FunctionName=vapocont  Parameters=PROPERTYTYPE, DEBUGLEVEL, MAXTOTALMESSAGES, MAXCONSECUTIVEMESSAGES,WRITETOFILE, FILENAME  SFunctionDeploymentMode=off  EnableBusSupport=off
  vapcont : Outport
  wires:
  SFunction/1 -> vapcont/1
  T/1 -> SFunction/3
  p/1 -> SFunction/4
  Fluid_Type/1 -> SFunction/1
  Fluid_Mix/1 -> SFunction/2
  value/1 -> SFunction/5

== system carnot/Basic/Material_Properties/Vapour_Pressure ==
  T : Inport
  p : Inport  Port=2
  Fluid_Type : Inport  Port=3
  Fluid_Mix : Inport  Port=4
  SFunction : S-Function  FunctionName=vappress  Parameters=DEBUGLEVEL,MAXTOTALMESSAGES,MAXCONSECUTIVEMESSAGES,WRITETOFILE,FILENAME  SFunctionDeploymentMode=off  EnableBusSupport=off
  vappress : Outport
  wires:
  SFunction/1 -> vappress/1
  T/1 -> SFunction/3
  p/1 -> SFunction/4
  Fluid_Type/1 -> SFunction/1
  Fluid_Mix/1 -> SFunction/2

== system carnot/Basic/Material_Properties/x2RelHum ==
  note: x · p
      | f =  -----------------
      |         ps ( RG/RD + x)
      |
      | RG = 287.1 Nm/kgK (Gas Constant Air)
      | RD = 461.5 Nm/kgK (Gas Constant Water Vapour)
      | x absolute Humudity
      | f relative Humidity
      | pD partial pressure of water vapour
  T : Inport
  p : Inport  Port=2
  x : Inport  Port=3
  Product1 : Product  Inputs=//**  SaturateOnIntegerOverflow=on  InputSameDT=on  OutDataTypeStr=Inherit: Same as first input
  Saturation : Saturate  UpperLimit=100  LowerLimit=0
  Sum : Sum  Inputs=|++  SaturateOnIntegerOverflow=on  InputSameDT=on  OutDataTypeStr=Inherit: Same as first input
  Vapour_Pressure : $bdroot/Basic/Material_Properties/Vapour_Pressure  VariantControl=CarlibClassic  INPUTARGUMENTS=state variables (classic)  DEBUGLEVEL=WARNINGLEVEL  MAXTOTALMESSAGES=inf  MAXCONSECUTIVEMESSAGES=inf  WRITETOFILE=0  FILENAME='errors.txt'
  mix : Constant  Value=0
  "molar mass fraction " : Constant  Value=287.1/461.5
  p12 : Constant
  to percent : Gain  Gain=100  SaturateOnIntegerOverflow=on  OutDataTypeStr=Inherit: Same as input  ParamDataTypeStr=Inherit: Same as input
  water : Constant
  rel_hum : Outport
  wires:
  mix/1 -> Vapour_Pressure/4
  p12/1 -> Vapour_Pressure/2
  water/1 -> Vapour_Pressure/3
  T/1 -> Vapour_Pressure/1
  Product1/1 -> to percent/1
  x/1 -> Sum/2, Product1/4
  p/1 -> Product1/3
  Sum/1 -> Product1/2
  Vapour_Pressure/1 -> Product1/1
  to percent/1 -> Saturation/1
  Saturation/1 -> rel_hum/1
  "molar mass fraction "/1 -> Sum/1

== system carnot/Basic/Pressure_Drop/Pressure_Drop ==
  THBin : Inport
  con : Inport  Port=2
  lin : Inport  Port=3
  qua : Inport  Port=4
  Bus Assignment : BusAssignment  AssignedSignals=Pressure,DPConstant,DPLinear,DPQuadratic
  Bus Selector1 : BusSelector  OutputSignals=Pressure
  Bus Selector2 : BusSelector  OutputSignals=ID
  Compare To Constant : simulink/Logic and Bit Operations/Compare To Constant  relop=>  const=10000  OutDataTypeStr=boolean
  Saturation : Saturate  UpperLimit=inf  LowerLimit=0
  calculate_dp : Subsystem
  sum1 : Sum  Inputs=+-  SaturateOnIntegerOverflow=on  InputSameDT=on  OutDataTypeStr=Inherit: Same as first input
  THB : Outport
  wires:
  Bus Selector2/1 -> Compare To Constant/1  "<ID>"
  Compare To Constant/1 -> calculate_dp/Enable
  calculate_dp/1(dp) -> sum1/2
  calculate_dp/4(qua) -> Bus Assignment/5
  calculate_dp/3(lin) -> Bus Assignment/4
  calculate_dp/2(con) -> Bus Assignment/3
  qua/1 -> calculate_dp/4(q)
  lin/1 -> calculate_dp/3(l)
  con/1 -> calculate_dp/2(c)
  Saturation/1 -> Bus Assignment/2
  Bus Selector1/1 -> sum1/1  "<Pressure>"
  Bus Assignment/1 -> THB/1  "THB"
  sum1/1 -> Saturation/1
  THBin/1 -> Bus Selector1/1, Bus Assignment/1, calculate_dp/1(THBin), Bus Selector2/1

== system carnot/Basic/Pressure_Drop/Pressure_Drop_Ceta ==
  THBin : Inport
  dp_coeff : Inport  Port=2
  Constant : Constant  Value=0
  Constant1 : Constant  Value=0
  Pressure_Drop : $bdroot/Basic/Pressure_Drop/Pressure_Drop
  pressuredropcoeff2clq : $bdroot/Basic/Pressure_Drop/pressuredropcoeff2clq
  THB : Outport
  wires:
  Pressure_Drop/1 -> THB/1
  THBin/1 -> pressuredropcoeff2clq/1, Pressure_Drop/1
  Constant/1 -> Pressure_Drop/2
  Constant1/1 -> Pressure_Drop/3
  pressuredropcoeff2clq/1 -> Pressure_Drop/4
  dp_coeff/1 -> pressuredropcoeff2clq/2

== system carnot/Basic/Pressure_Drop/Pressure_Drop_Collector ==
  Tnodes : Inport
  THBin : Inport  Port=2
  position : Inport  Port=3
  Bus Selector3 : BusSelector  OutputSignals=inclination
  Degrees to Radians : simulink_extras/Transformations/Degrees to Radians
  Gain : Gain  Gain=len
  Pressure_Drop_Fix : $bdroot/Basic/Pressure_Drop/Pressure_Drop_Fix  con=0  lin=lin  qua=qua
  Pressure_Drop_staticHeight : $bdroot/Basic/Pressure_Drop/Pressure_Drop_staticHeight
  Trigonometric Function : Trigonometry
  THB : Outport
  wires:
  Degrees to Radians/1 -> Trigonometric Function/1
  Pressure_Drop_staticHeight/1 -> THB/1
  Tnodes/1 -> Pressure_Drop_staticHeight/1
  Pressure_Drop_Fix/1 -> Pressure_Drop_staticHeight/2
  THBin/1 -> Pressure_Drop_Fix/1
  Trigonometric Function/1 -> Gain/1
  position/1 -> Bus Selector3/1
  Bus Selector3/1 -> Degrees to Radians/1  "<inclination>"
  Gain/1 -> Pressure_Drop_staticHeight/3

== system carnot/Basic/Pressure_Drop/Pressure_Drop_Fix ==
  THB : Inport
  Bus Assignment1 : BusAssignment  AssignedSignals=Pressure,DPConstant,DPLinear,DPQuadratic
  Bus Selector3 : BusSelector  OutputSignals=MassFlow,Pressure
  Bus Selector4 : BusSelector  OutputSignals=DPConstant,DPLinear,DPQuadratic  OutputAsBus=on
  Constant : Constant  Value=lin
  Constant1 : Constant  Value=qua
  Constant2 : Constant  Value=con
  Demux2 : Demux  Outputs=3
  Pressuredrop : $bdroot/Basic/Pressure_Drop/Pressuredrop
  Terminator1 : Terminator
  THB_ : Outport
  wires:
  Pressuredrop/3 -> Terminator1/1
  THB/1 -> Bus Assignment1/1, Bus Selector4/1, Bus Selector3/1
  Bus Assignment1/1 -> THB_/1
  Demux2/1 -> Bus Assignment1/3
  Demux2/2 -> Bus Assignment1/4
  Demux2/3 -> Bus Assignment1/5
  Bus Selector3/1 -> Pressuredrop/1  "<MassFlow>"
  Bus Selector3/2 -> Pressuredrop/2  "<Pressure>"
  Bus Selector4/1 -> Pressuredrop/3
  Constant2/1 -> Pressuredrop/4
  Constant/1 -> Pressuredrop/5
  Constant1/1 -> Pressuredrop/6
  Pressuredrop/1 -> Bus Assignment1/2
  Pressuredrop/2 -> Demux2/1

== system carnot/Basic/Pressure_Drop/Pressure_Drop_PipeTheory ==
  Tnodes : Inport
  THBin : Inport  Port=2
  Abs : Abs
  Bus Assignment : BusAssignment  AssignedSignals=Pressure,DPConstant,DPLinear,DPQuadratic
  Bus Selector : BusSelector  OutputSignals=MassFlow,Pressure
  Bus Selector1 : BusSelector  OutputSignals=DPConstant,DPLinear,DPQuadratic  OutputAsBus=on
  Bus Selector2 : BusSelector  OutputSignals=ID
  Compare To Constant1 : simulink/Logic and Bit Operations/Compare To Constant  relop=>  const=10000  OutDataTypeStr=boolean
  DP_Geometry : Subsystem
  Demux : Demux  Outputs=3
  Pressuredrop : $bdroot/Basic/Pressure_Drop/Pressuredrop
  Terminator : Terminator
  Terminator1 : Terminator
  const1 : Constant  Value=0
  THB : Outport
  wires:
  DP_Geometry/3(dp) -> Terminator1/1
  DP_Geometry/2(qua) -> Pressuredrop/6
  DP_Geometry/1(lin) -> Pressuredrop/5
  Pressuredrop/2 -> Demux/1
  Demux/3 -> Bus Assignment/5
  Demux/2 -> Bus Assignment/4
  Demux/1 -> Bus Assignment/3
  Pressuredrop/1 -> Bus Assignment/2
  Bus Assignment/1 -> THB/1
  THBin/1 -> Bus Selector/1, Bus Selector1/1, Bus Selector2/1, DP_Geometry/2(mdot), Bus Assignment/1
  Abs/1 -> Compare To Constant1/1
  Bus Selector1/1 -> Pressuredrop/3
  Bus Selector/1 -> Pressuredrop/1  "<MassFlow>"
  Bus Selector/2 -> Pressuredrop/2  "<Pressure>"
  Bus Selector2/1 -> Abs/1  "<ID>"
  Tnodes/1 -> DP_Geometry/1(Tnodes)
  Compare To Constant1/1 -> DP_Geometry/Enable
  Pressuredrop/3 -> Terminator/1
  const1/1 -> Pressuredrop/4

== system carnot/Basic/Pressure_Drop/Pressure_Drop_StorageHX ==
  THBin : Inport
  Bus Selector : BusSelector  OutputSignals=Temperature
  Constant : Constant  Value=hgt
  Pressure_Drop_Fix : $bdroot/Basic/Pressure_Drop/Pressure_Drop_Fix  con=0  lin=dplin  qua=dpqua
  Pressure_Drop_changeD : $bdroot/Basic/Pressure_Drop/Pressure_Drop_changeD  dia=dia
  Pressure_Drop_staticHeight : $bdroot/Basic/Pressure_Drop/Pressure_Drop_staticHeight
  THB : Outport
  wires:
  Pressure_Drop_staticHeight/1 -> Pressure_Drop_Fix/1
  Pressure_Drop_changeD/1 -> Pressure_Drop_staticHeight/2
  Constant/1 -> Pressure_Drop_staticHeight/3
  THBin/1 -> Pressure_Drop_changeD/1, Bus Selector/1
  Bus Selector/1 -> Pressure_Drop_staticHeight/1  "<Temperature>"
  Pressure_Drop_Fix/1 -> THB/1

== system carnot/Basic/Pressure_Drop/Pressure_Drop_StoragePipe ==
  Tnodes : Inport
  THBin : Inport  Port=2
  Constant : Constant  Value=hgt
  Pressure_Drop_changeD : $bdroot/Basic/Pressure_Drop/Pressure_Drop_changeD  dia=dpipe
  Pressure_Drop_decreaseD : $bdroot/Basic/Pressure_Drop/Pressure_Drop_changeD  dia=dpipe
  Pressure_Drop_increaseD : $bdroot/Basic/Pressure_Drop/Pressure_Drop_changeD  dia=dstg
  Pressure_Drop_staticHeight : $bdroot/Basic/Pressure_Drop/Pressure_Drop_staticHeight
  THB : Outport
  wires:
  THBin/1 -> Pressure_Drop_changeD/1
  Constant/1 -> Pressure_Drop_staticHeight/3
  Pressure_Drop_increaseD/1 -> Pressure_Drop_decreaseD/1
  Tnodes/1 -> Pressure_Drop_staticHeight/1
  Pressure_Drop_staticHeight/1 -> THB/1
  Pressure_Drop_decreaseD/1 -> Pressure_Drop_staticHeight/2
  Pressure_Drop_changeD/1 -> Pressure_Drop_increaseD/1

== system carnot/Basic/Pressure_Drop/Pressure_Drop_changeD ==
  THBin : Inport
  2/pi/d^2/density : Subsystem
  Abs : Abs
  Bus Assignment : BusAssignment  AssignedSignals=Pressure,DPConstant,DPLinear,DPQuadratic,DiameterLastPiece
  Bus Selector : BusSelector  OutputSignals=MassFlow,Pressure
  Bus Selector1 : BusSelector  OutputSignals=DPConstant,DPLinear,DPQuadratic  OutputAsBus=on
  Bus Selector2 : BusSelector  OutputSignals=ID
  Compare To Constant1 : simulink/Logic and Bit Operations/Compare To Constant  relop=>  const=10000  OutDataTypeStr=boolean
  Constant : Constant  Value=0
  Demux : Demux  Outputs=3
  Pressuredrop : $bdroot/Basic/Pressure_Drop/Pressuredrop
  Terminator : Terminator
  diameter : Constant  Value=dia
  THB : Outport
  wires:
  diameter/1 -> Bus Assignment/6
  Pressuredrop/2 -> Demux/1
  Demux/3 -> Bus Assignment/5
  Demux/2 -> Bus Assignment/4
  Demux/1 -> Bus Assignment/3
  Pressuredrop/1 -> Bus Assignment/2
  Bus Assignment/1 -> THB/1
  THBin/1 -> Bus Assignment/1, Bus Selector/1, Bus Selector1/1, Bus Selector2/1, 2/pi/d^2/density/1(THB)
  Abs/1 -> Compare To Constant1/1
  Bus Selector1/1 -> Pressuredrop/3
  Bus Selector/1 -> Pressuredrop/1  "<MassFlow>"
  Bus Selector/2 -> Pressuredrop/2  "<Pressure>"
  Bus Selector2/1 -> Abs/1  "<ID>"
  Constant/1 -> Pressuredrop/5, Pressuredrop/4
  2/pi/d^2/density/1(qua) -> Pressuredrop/6
  Compare To Constant1/1 -> 2/pi/d^2/density/Enable
  Pressuredrop/3 -> Terminator/1

== system carnot/Basic/Pressure_Drop/Pressure_Drop_staticHeight ==
  Tnodes : Inport
  THBin : Inport  Port=2
  height : Inport  Port=3
  Abs : Abs
  Bus Assignment : BusAssignment  AssignedSignals=Pressure,DPConstant,DPLinear,DPQuadratic,GeodeticHeight
  Bus Selector : BusSelector  OutputSignals=MassFlow,Pressure
  Bus Selector1 : BusSelector  OutputSignals=DPConstant,DPLinear,DPQuadratic  OutputAsBus=on
  Bus Selector2 : BusSelector  OutputSignals=ID
  Compare To Constant : simulink/Logic and Bit Operations/Compare To Constant  relop=>  const=20000  OutDataTypeStr=boolean
  Demux : Demux  Outputs=3
  Density_x_Gravity : Subsystem
  Pressuredrop : $bdroot/Basic/Pressure_Drop/Pressuredrop
  Terminator : Terminator
  const1 : Constant  Value=0
  const2 : Constant  Value=0
  THB : Outport
  wires:
  Density_x_Gravity/2(GeodeticHeight) -> Bus Assignment/6
  height/1 -> Density_x_Gravity/3(height)
  Pressuredrop/2 -> Demux/1
  Demux/3 -> Bus Assignment/5
  Demux/2 -> Bus Assignment/4
  Demux/1 -> Bus Assignment/3
  Pressuredrop/1 -> Bus Assignment/2
  Bus Assignment/1 -> THB/1
  THBin/1 -> Bus Assignment/1, Bus Selector/1, Bus Selector1/1, Density_x_Gravity/2(THB), Bus Selector2/1
  Abs/1 -> Compare To Constant/1
  Bus Selector1/1 -> Pressuredrop/3
  Bus Selector/1 -> Pressuredrop/1  "<MassFlow>"
  Bus Selector/2 -> Pressuredrop/2  "<Pressure>"
  Bus Selector2/1 -> Abs/1  "<ID>"
  Tnodes/1 -> Density_x_Gravity/1(Tnodes)
  Compare To Constant/1 -> Density_x_Gravity/Enable
  Density_x_Gravity/1(pstat) -> Pressuredrop/4
  Pressuredrop/3 -> Terminator/1
  const1/1 -> Pressuredrop/5
  const2/1 -> Pressuredrop/6

== system carnot/Basic/Pressure_Drop/Pressuredrop ==
  note: no pressure below 0 Pa
  mdot : Inport
  p_in : Inport  Port=2
  clq_in : Inport  Port=3
  con : Inport  Port=4
  lin : Inport  Port=5
  qua : Inport  Port=6
  Constant : Constant
  Dot Product : DotProduct  InputSameDT=on  OutDataTypeStr=Inherit: Inherit via internal rule
  Math Function : Math  Operator=square  SaturateOnIntegerOverflow=on
  Mux : Mux  Inputs=3
  Mux1 : Mux  Inputs=3
  Saturation : Saturate  UpperLimit=inf  LowerLimit=0
  sum : Sum  SaturateOnIntegerOverflow=on  InputSameDT=on  OutDataTypeStr=Inherit: Same as first input
  sum1 : Sum  Inputs=+-  SaturateOnIntegerOverflow=on  InputSameDT=on  OutDataTypeStr=Inherit: Same as first input
  p_out : Outport
  clq_out : Outport  Port=2
  dp : Outport  Port=3
  wires:
  sum1/1 -> Saturation/1
  p_in/1 -> sum1/1
  Dot Product/1 -> dp/1, sum1/2
  Mux1/1 -> Dot Product/2, sum/2
  sum/1 -> clq_out/1
  clq_in/1 -> sum/1
  qua/1 -> Mux1/3
  lin/1 -> Mux1/2
  con/1 -> Mux1/1
  Mux/1 -> Dot Product/1
  Math Function/1 -> Mux/3
  mdot/1 -> Math Function/1, Mux/2
  Constant/1 -> Mux/1
  Saturation/1 -> p_out/1

== system carnot/Basic/Pressure_Drop/clq2friction_coeff ==
  note: dp = lambda * l * rho / (dia * 2) * v^2
      |    = lambda * l * rho / (dia * 2) * vdot^2 / A^2
      |     = lambda * l * rho / (dia * 2) * mdot^2 / rho^2 / A^2
      |     = lambda * l / (dia * 2) * mdot^2 / rho / A^2
      |     = lambda * l / (dia * 2) * mdot^2 / rho / (pi*(dia/2)^2)^2
      |     = 8 * lambda * l * mdot^2 / (rho * pi^2 * dia^5)
      |
      | dp = c + l*mdot + q*mdot^2
      |
      | -> lambda = q * rho * pi^2 * dia^5 / (8 * l)
      | c = 0; l = 0;
  THB : Inport
  q : Inport  Port=2
  Constant1 : Constant  Value=8
  Constant2 : Constant  Value=5
  Density : $bdroot/Basic/Material_Properties/Density  VariantControl=CarlibClassic  INPUTARGUMENTS=THB  DEBUGLEVEL=DEBUGLEVEL  MAXTOTALWARNINGS=inf  MAXCONSECUTIVEWARNINGS=inf  WRITETOFILE=0  FILENAME='errors.txt'
  Gain : Gain  Gain=pi^2
  Math Function1 : Math  Operator=pow  SaturateOnIntegerOverflow=on
  Product : Product  Inputs=**/*  RndMeth=Zero
  diameter : Constant  Value=Value
  length : Gain  Gain=Gain
  pipe_friction_coeff : Outport
  wires:
  Product/1 -> pipe_friction_coeff/1
  Gain/1 -> Product/1
  THB/1 -> Density/1
  Density/1 -> Gain/1
  Math Function1/1 -> Product/2
  diameter/1 -> Math Function1/1
  Constant2/1 -> Math Function1/2
  length/1 -> Product/3
  Constant1/1 -> length/1
  q/1 -> Product/4

== system carnot/Basic/Pressure_Drop/clq2pressuredropcoeff ==
  note: dp = zeta * density/2 * w^2
      | dp = c + l*mdot + q*mdot^2    Carnot approach (here c = l = 0)
      | with mdot = Vdot*density = w*A*density  -> w = mdot/A/density
      | dp = zeta * density/2 * mdot^2/A^2/density^2
      | dp = zeta/(2*A^2*density) * mdot^2
      | -> q = zeta/(2*A^2*density)
      | with A = pi/4*d^2
      | -> q = 8*zeta / (pi^2*d^4*density)
      | -> zeta = q * pi^2*d^4*density / 8
  THB : Inport
  q : Inport  Port=2
  Bus Selector3 : BusSelector  OutputSignals=DiameterLastPiece
  Density : $bdroot/Basic/Material_Properties/Density  VariantControl=CarlibClassic  INPUTARGUMENTS=THB  DEBUGLEVEL=DEBUGLEVEL  MAXTOTALWARNINGS=inf  MAXCONSECUTIVEWARNINGS=inf  WRITETOFILE=0  FILENAME='errors.txt'
  Gain : Gain  Gain=pi^2
  Gain1 : Gain  Gain=1/8
  Math Function1 : Math  Operator=square  SaturateOnIntegerOverflow=on
  Math Function4 : Math  Operator=square  SaturateOnIntegerOverflow=on
  Product : Product  Inputs=3  RndMeth=Zero
  dp_coeff : Outport
  wires:
  Product/1 -> dp_coeff/1
  Gain/1 -> Product/1
  THB/1 -> Density/1, Bus Selector3/1
  Density/1 -> Gain/1
  Bus Selector3/1 -> Math Function1/1  "<DiameterLastPiece>"
  Math Function1/1 -> Math Function4/1
  Math Function4/1 -> Product/2
  q/1 -> Gain1/1
  Gain1/1 -> Product/3

== system carnot/Basic/Pressure_Drop/friction_coeff2clq ==
  note: dp = lambda * l * rho / (dia * 2) * v^2
      |    = lambda * l * rho / (dia * 2) * vdot^2 / A^2
      |     = lambda * l * rho / (dia * 2) * mdot^2 / rho^2 / A^2
      |     = lambda * l / (dia * 2) * mdot^2 / rho / A^2
      |     = lambda * l / (dia * 2) * mdot^2 / rho / (pi*(dia/2)^2)^2
      |     = 8 * lambda * l * mdot^2 / (rho * pi^2 * dia^5)
      |
      | dp = c + l*mdot + q*mdot^2
      |
      | -> q = 8 * lambda * l / (rho * pi^2 * dia^5)
      | c = 0; l = 0;
  THB : Inport
  pipe_friction_coeff : Inport  Port=2
  Constant2 : Constant  Value=5
  Density : $bdroot/Basic/Material_Properties/Density  VariantControl=CarlibClassic  INPUTARGUMENTS=THB  DEBUGLEVEL=DEBUGLEVEL  MAXTOTALWARNINGS=inf  MAXCONSECUTIVEWARNINGS=inf  WRITETOFILE=0  FILENAME='errors.txt'
  Gain : Gain  Gain=pi^2
  Gain1 : Gain  Gain=8
  Math Function1 : Math  Operator=pow  SaturateOnIntegerOverflow=on
  Product : Product  Inputs=//*  RndMeth=Zero
  diameter : Constant  Value=Value
  length : Gain  Gain=Gain
  q : Outport
  wires:
  Product/1 -> q/1
  Gain/1 -> Product/1
  THB/1 -> Density/1
  Density/1 -> Gain/1
  Math Function1/1 -> Product/2
  pipe_friction_coeff/1 -> Gain1/1
  Gain1/1 -> length/1
  diameter/1 -> Math Function1/1
  Constant2/1 -> Math Function1/2
  length/1 -> Product/3

== system carnot/Basic/Pressure_Drop/pressuredropcoeff2clq ==
  note: dp = zeta * density/2 * w^2
      | dp = c + l*mdot + q*mdot^2    Carnot approach (here c = l = 0)
      | with mdot = Vdot*density = w*A*density  -> w = mdot/A/density
      | dp = zeta * density/2 * mdot^2/A^2/density^2
      | dp = zeta/(2*A^2*density) * mdot^2
      | -> q = zeta/(2*A^2*density)
      | with A = pi/4*d^2
      | -> q = 8*zeta / (pi^2*d^4*density)
  THB : Inport
  dp_coeff : Inport  Port=2
  Bus Selector3 : BusSelector  OutputSignals=DiameterLastPiece
  Density : $bdroot/Basic/Material_Properties/Density  VariantControl=CarlibClassic  INPUTARGUMENTS=THB  DEBUGLEVEL=DEBUGLEVEL  MAXTOTALWARNINGS=inf  MAXCONSECUTIVEWARNINGS=inf  WRITETOFILE=0  FILENAME='errors.txt'
  Gain : Gain  Gain=pi^2
  Gain1 : Gain  Gain=8
  Math Function1 : Math  Operator=square  SaturateOnIntegerOverflow=on
  Math Function4 : Math  Operator=square  SaturateOnIntegerOverflow=on
  Product : Product  Inputs=//*  RndMeth=Zero
  q : Outport
  wires:
  Product/1 -> q/1
  Gain/1 -> Product/1
  THB/1 -> Density/1, Bus Selector3/1
  Density/1 -> Gain/1
  Bus Selector3/1 -> Math Function1/1  "<DiameterLastPiece>"
  Math Function1/1 -> Math Function4/1
  Math Function4/1 -> Product/2
  dp_coeff/1 -> Gain1/1
  Gain1/1 -> Product/3

== system carnot/Basic/Pressure_Drop/relFlowCoeff2qua ==
  note: The definition of the flow coefficient Kv is:
      | Kv = Vdot * sqrt(1e5Pa/dp * density/1000kg/m³)
      | Vdot is the volumetric flow rate in m³/h
      | resolve equation for pressure drop dp:
      | (Kv/Vdot)² = 1e5Pa/dp * density/1000kg/m³
      | dp = (1e5/1000 Pa*m³/kg) * density * (Vdot/Kv)²
      | dp = (100 Pa*m³/kg) * density * (Vdot/Kv)²
      | with Vdot = mdot/density
      | dp = (100 Pa*m³/kg)/density * (mdot/Kv)²
      | change unit of Kv: kg/h = kg/(3600s)
      | dp = (100 Pa*m³/kg) * (3600 s/h)² / density * (mdot/Kv)²
      | Carnot equation: dp = qua * mdot²
      | qua = (100 Pa*m³/kg) * (3600 s/h)² / (density*Kv²)
  THB : Inport
  psi : Inport  Port=2
  Constant : Constant  Value=3600^2*100
  Density : $bdroot/Basic/Material_Properties/Density  VariantControl=CarlibClassic  INPUTARGUMENTS=THB  DEBUGLEVEL=DEBUGLEVEL  MAXTOTALWARNINGS=inf  MAXCONSECUTIVEWARNINGS=inf  WRITETOFILE=0  FILENAME='errors.txt'
  Kvs : Gain  Gain=kvs
  Math Function : Math  Operator=square  SaturateOnIntegerOverflow=on
  Product1 : Product  Inputs=*//
  qua : Outport
  wires:
  THB/1 -> Density/1
  Density/1 -> Product1/3
  Math Function/1 -> Product1/2
  Product1/1 -> qua/1
  Constant/1 -> Product1/1
  psi/1 -> Kvs/1
  Kvs/1 -> Math Function/1  "Kv"

== system carnot/Basic/Thermal_Models/Combustion_Calculation ==
  Qdot_fuel : Inport
  efficiency : Inport  Port=2
  Pelec : Inport  Port=3
  Tm : Inport  Port=4
  fuel : Inport  Port=5
  Enable : EnablePort
  Bus Creator : BusCreator  Inputs=16
  Bus Selector : BusSelector  OutputSignals=Fuel_ID,Pressure,h_Vector,Price,MassFraction_H,MassFraction_C,MassFraction_O,MassFraction_S,MassFraction_N,MassFraction_H2O
  Selector : Selector  IndexOptions=Index vector (dialog)  Indices=[1]  OutputSizes=1
  Signal Conversion : SignalConversion  OverrideOpt=off
  exhaust gas : Subsystem
  mdotCO2 : Product  SaturateOnIntegerOverflow=on  InputSameDT=on  OutDataTypeStr=Inherit: Same as first input
  mdotH20 : Product  SaturateOnIntegerOverflow=on  InputSameDT=on  OutDataTypeStr=Inherit: Same as first input
  mdotN2 : Product  SaturateOnIntegerOverflow=on  InputSameDT=on  OutDataTypeStr=Inherit: Same as first input
  mdotNOx : Product  SaturateOnIntegerOverflow=on  InputSameDT=on  OutDataTypeStr=Inherit: Same as first input
  mdotSO2 : Product  SaturateOnIntegerOverflow=on  InputSameDT=on  OutDataTypeStr=Inherit: Same as first input
  mdot_CO : Constant  Value=0
  mdot_CxHy : Constant  Value=0
  mdot_O2 : Constant  Value=0
  n2 : Constant  Value=0
  pricedot : Product  SaturateOnIntegerOverflow=on  InputSameDT=on  OutDataTypeStr=Inherit: Same as first input
  prod : Product  Inputs=*/  SaturateOnIntegerOverflow=on  InputSameDT=on  OutDataTypeStr=Inherit: Same as first input
  eco : Outport  InitialOutput=0
  wires:
  Tm/1 -> Bus Creator/2  "Tmean"
  Qdot_fuel/1 -> Bus Creator/5, prod/1  "Qdot_fuel"
  mdotN2/1 -> Bus Creator/12  "mdotN2"
  exhaust gas/2(H2O) -> mdotH20/2
  exhaust gas/1(CO2) -> mdotCO2/2
  exhaust gas/4(N2) -> mdotN2/2
  n2/1 -> mdotNOx/2
  exhaust gas/3(SO2) -> mdotSO2/2
  Bus Selector/10 -> exhaust gas/7(w)  "<MassFraction_H2O>"
  Bus Selector/9 -> exhaust gas/6(n)  "<MassFraction_N>"
  Bus Selector/8 -> exhaust gas/5(s)  "<MassFraction_S>"
  Bus Selector/7 -> exhaust gas/4(o)  "<MassFraction_O>"
  Bus Selector/6 -> exhaust gas/3(c)  "<MassFraction_C>"
  Bus Selector/5 -> exhaust gas/2(h)  "<MassFraction_H>"
  Bus Selector/2 -> Bus Creator/4  "<Pressure>"
  Bus Selector/1 -> Bus Creator/1, exhaust gas/1(ID)  "<Fuel_ID>"
  prod/1 -> Bus Creator/3, mdotN2/1, mdotNOx/1, mdotSO2/1, mdotCO2/1, mdotH20/1, pricedot/1  "mdot_fuel"
  Bus Selector/4 -> pricedot/2  "<Price>"
  mdot_CxHy/1 -> Bus Creator/15  "mdot_CxHy"
  mdot_CO/1 -> Bus Creator/14  "mdot_CO"
  mdotNOx/1 -> Bus Creator/13  "mdotNOx"
  mdotSO2/1 -> Bus Creator/11  "mdotSO2"
  mdot_O2/1 -> Bus Creator/10  "mdot_O2"
  mdotCO2/1 -> Bus Creator/9  "mdotCO2"
  mdotH20/1 -> Bus Creator/8  "mdotH20"
  pricedot/1 -> Bus Creator/7  "MoneyFlow"
  Pelec/1 -> Bus Creator/6  "Pelec"
  Bus Creator/1 -> Signal Conversion/1
  Bus Selector/3 -> Selector/1  "<h_Vector>"
  fuel/1 -> Bus Selector/1
  efficiency/1 -> Bus Creator/16  "Efficiency"
  Selector/1 -> prod/2
  Signal Conversion/1 -> eco/1
